simulink model "ArrayTruncation"  (R2015a)
settings: Solver=ode45  StartTime=0.0  StopTime=10.0  RelTol=1e-3
undefined symbols (not defined in the file): gray, Rec, SDTV
libraries: visionconversions x1, visionanalysis x1, dspvision x1, visionsinks x1
settings Model: Creator=hoanga  LastModifiedBy=hoanga

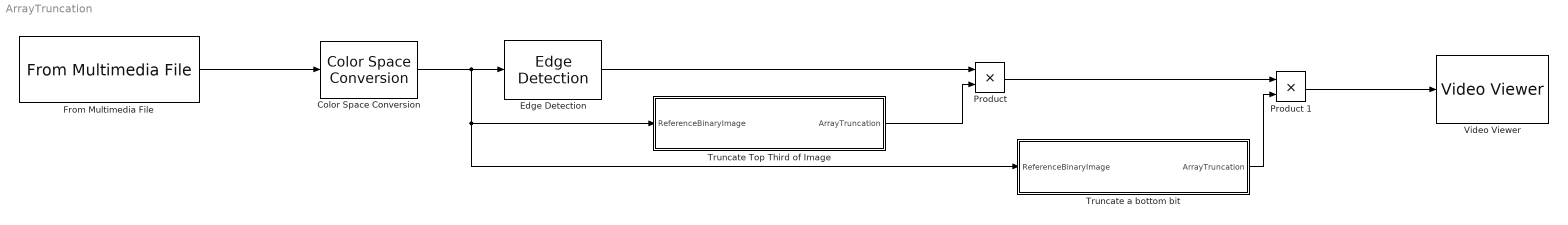
== system ArrayTruncation ==
  Color Space Conversion : visionconversions/Color Space  Conversion  conversion=Obsolete  conversionActive=R'G'B' to intensity  wp_str=D65  rec=Rec. 601 (SDTV)  sys=1125/60/2:1  imagePorts=One multidimensional signal
  Edge Detection : visionanalysis/Edge Detection  method=Sobel  outputType=Binary image  userDefinedThreshold=off  thresholdSource=Input port  threshold=20  thresholdTuning=4  edgeThinning=off  threshold_canny=[0.25 0.60]  autoPercent=70  sigma=1  prodOutputMode=Binary point scaling  prodOutputWordLength=32  prodOutputFracLength=8  roundingMode=Floor  overflowMode=off
  From Multimedia File : dspvision/From Multimedia File  inputFilename=C:\Users\hoanga\Desktop\Video.mp4  loop=on  numPlays=inf  outputStreams=Video only  videoDataType=single  audioDataType=int16  inheritSampleTime=on  userDefinedSampleTime=1/30  noAudioOutput=off  isIntensityVideo=off  fourcc=RGB  colorVideoFormat=One multidimensional signal  outputEOF=off  dataOrg=Column-major  audioFrameSize=1024  computeAudioFrameSize=off  outSamplingMode=Sample based
  "Product " : Product
  Product 1 : Product
  Truncate Top Third of Image : MATLAB Function  TreatAsAtomicUnit=on
  Truncate a bottom bit : MATLAB Function  TreatAsAtomicUnit=on
  Video Viewer : visionsinks/Video Viewer  inputType=Obsolete7b  imagePorts=One multidimensional signal  useColorMap=off  colormapValue=gray(256)  specRange=off  minInputVal=0  maxInputVal=255  FigPos=[1921 1038 1920 939]  AxisZoom=on  trueSizedOnce=off  OpenAtMdlStart=on  DefaultConfigurationName=vipscopes.VideoViewerScopeCfg
  wires:
  Color Space Conversion/1 -> Truncate a bottom bit/1(ReferenceBinaryImage), Truncate Top Third of Image/1(ReferenceBinaryImage), Edge Detection/1
  From Multimedia File/1 -> Color Space Conversion/1
  Truncate Top Third of Image/1(ArrayTruncation) -> "Product "/2
  Edge Detection/1 -> "Product "/1
  "Product "/1 -> Product 1/1
  Truncate a bottom bit/1(ArrayTruncation) -> Product 1/2
  Product 1/1 -> Video Viewer/1

== matlab function ArrayTruncation/Truncate a bottom bit ==
  data: ReferenceBinaryImage input; ArrayTruncation output
function ArrayTruncation = fcn(ReferenceBinaryImage)

%This function truncates the image you are processing by O variable fraction.
% In this case, O was set to 3 and deletes the first third of the flattened
% 2D array.

O = 9/10;

[x,y] = size(ReferenceBinaryImage);
matrix = ones(x, y);

for i = x*O:x
    for j = 1:y
        matrix(i,j) = 0;
    end
end

ArrayTruncation = matrix;

end

== matlab function ArrayTruncation/Truncate Top Third of Image ==
  data: ReferenceBinaryImage input; ArrayTruncation output
function ArrayTruncation = fcn(ReferenceBinaryImage)

%This function truncates the image you are processing by O variable fraction.
% In this case, O was set to 3 and deletes the first third of the flattened
% 2D array.

O = 3;

[x,y] = size(ReferenceBinaryImage);
matrix = zeros(x, y);

for i = x/O:x
    for j = 1:y
        matrix(i,j) = 1;
    end
end

ArrayTruncation = matrix;

end
